simulink model "seguimiento_lmi"  (R2021a)
settings: Solver=VariableStepAuto  StartTime=0.0  StopTime=10.0  RelTol=1e-3
settings Model: Creator=jmata  LastModifiedBy=jmata

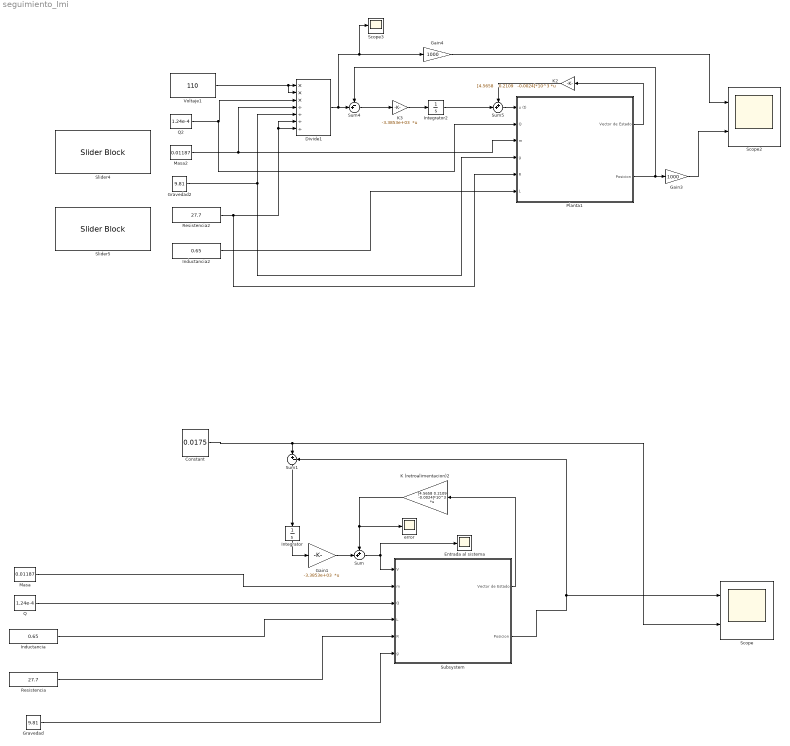
== system seguimiento_lmi ==
  Constant : Constant  Value=0.0175
  Divide1 : Product  Inputs=***////
  Entrada al sistema : Scope
  Gain1 : Gain  Gain=-3.3853e+03  Multiplication=Matrix(K*u)
  Gain3 : Gain  Gain=1000
  Gain4 : Gain  Gain=1000
  Gravedad : Constant  Value=9.81
  Gravedad2 : Constant  Value=9.81
  Inductancia : Constant  Value=0.65  VectorParams1D=off
  Inductancia2 : Constant  Value=0.65
  Integrator : Integrator
  Integrator2 : Integrator
  K (retroalimentacion)2 : Gain  Gain="[4.5658    0.2109   -0.0024]*10^3"  Multiplication=Matrix(K*u)
  K2 : Gain  Gain="[4.5658    0.2109   -0.0024]*10^3"  Multiplication=Matrix(K*u)
  K3 : Gain  Gain=-3.3853e+03  Multiplication=Matrix(K*u)
  Masa : Constant  Value=0.01187
  Masa2 : Constant  Value=0.01187
  Planta1 : Subsystem
  Q : Constant  Value=1.24e-4
  Q2 : Constant  Value=1.24e-4
  Resistencia : Constant  Value=27.7
  Resistencia2 : Constant  Value=27.7
  Scope : Scope  NumInputPorts=2
  Scope2 : Scope  NumInputPorts=2
  Scope3 : Scope
  Slider4 : SliderBlock  ScaleMin=25  ScaleMax=30
  Slider5 : SliderBlock  ScaleMin=0.585  ScaleMax=0.715
  Subsystem : Subsystem
  Sum : Sum  Inputs=++|
  Sum1 : Sum  Inputs=|+-
  Sum4 : Sum  Inputs=-+|
  Sum5 : Sum  Inputs=++|
  Voltaje1 : Constant  Value=110
  error : Scope
  wires:
  Constant/1 -> Scope/2, Sum1/1
  Gravedad/1 -> Subsystem/6(g)
  Masa/1 -> Subsystem/2(m)
  Inductancia/1 -> Subsystem/4(L)
  Sum1/1 -> Integrator/1
  Gain1/1 -> Sum/2
  Integrator/1 -> Gain1/1
  Resistencia/1 -> Subsystem/5(R)
  Subsystem/2(Posicion) -> Sum1/2, Scope/1
  Sum/1 -> Subsystem/1(V), Entrada al sistema/1
  Q/1 -> Subsystem/3(Q)
  Subsystem/1(Vector de Estado) -> K (retroalimentacion)2/1
  K (retroalimentacion)2/1 -> Sum/1, error/1
  Gain4/1 -> Scope2/1
  Divide1/1 -> Sum4/2, Scope3/1, Gain4/1
  Q2/1 -> Planta1/2(Q), Divide1/3
  Gravedad2/1 -> Divide1/5, Planta1/4(g)
  Gain3/1 -> Scope2/2
  Voltaje1/1 -> Divide1/2, Divide1/1
  Sum5/1 -> Planta1/1(u (t))
  Planta1/2(Posicion) -> Gain3/1, Sum4/1
  Masa2/1 -> Planta1/3(m), Divide1/4
  Planta1/1(Vector de Estado) -> K2/1
  Sum4/1 -> K3/1
  K2/1 -> Sum5/1
  K3/1 -> Integrator2/1
  Resistencia2/1 -> Divide1/7, Divide1/6, Planta1/5(R)
  Integrator2/1 -> Sum5/2
  Inductancia2/1 -> Planta1/6(L)

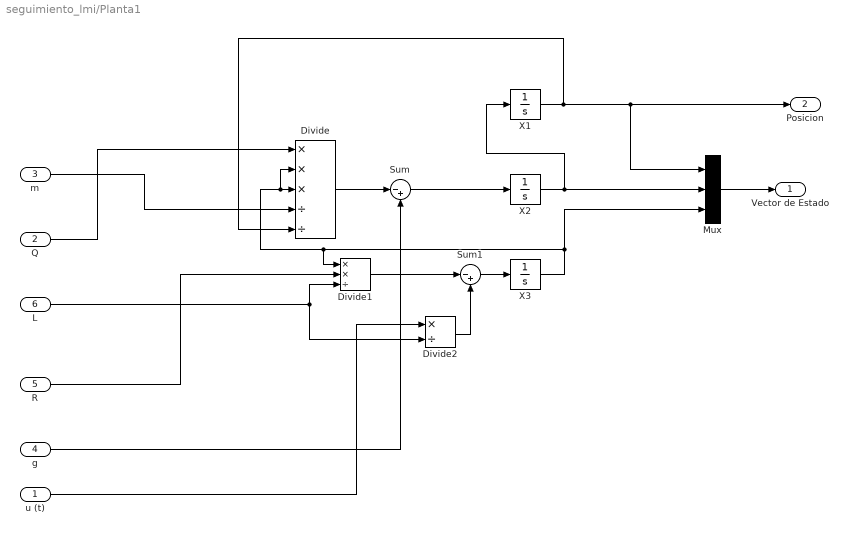
== system seguimiento_lmi/Planta1 ==
  u (t) : Inport
  Q : Inport  Port=2
  m : Inport  Port=3
  g : Inport  Port=4
  R : Inport  Port=5
  L : Inport  Port=6
  Divide : Product  Inputs=***//
  Divide1 : Product  Inputs=**/
  Divide2 : Product  Inputs=*/
  Mux : Mux  Inputs=3
  Sum : Sum  Inputs=|-+
  Sum1 : Sum  Inputs=|-+
  X1 : Integrator  InitialCondition=14.79e-3
  X2 : Integrator
  X3 : Integrator  InitialCondition=110/27.7
  Vector de Estado : Outport
  Posicion : Outport  Port=2
  wires:
  Divide/1 -> Sum/1
  Sum/1 -> X2/1
  L/1 -> Divide2/2, Divide1/3
  Sum1/1 -> X3/1
  X3/1 -> Mux/3, Divide1/1, Divide/2, Divide/3
  Divide2/1 -> Sum1/2
  X1/1 -> Posicion/1, Mux/1, Divide/5
  X2/1 -> Mux/2, X1/1
  g/1 -> Sum/2
  Divide1/1 -> Sum1/1
  m/1 -> Divide/4
  Q/1 -> Divide/1
  Mux/1 -> Vector de Estado/1
  R/1 -> Divide1/2
  u (t)/1 -> Divide2/1

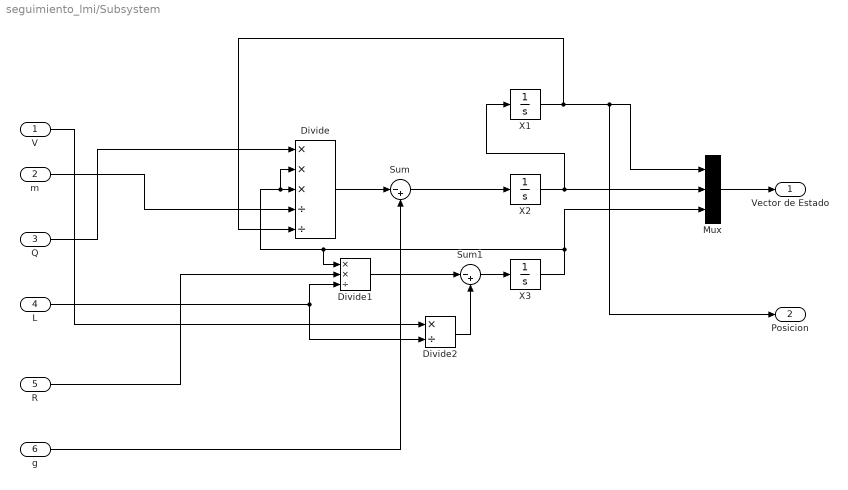
== system seguimiento_lmi/Subsystem ==
  V : Inport
  m : Inport  Port=2
  Q : Inport  Port=3
  L : Inport  Port=4
  R : Inport  Port=5
  g : Inport  Port=6
  Divide : Product  Inputs=***//
  Divide1 : Product  Inputs=**/
  Divide2 : Product  Inputs=*/
  Mux : Mux  Inputs=3
  Sum : Sum  Inputs=|-+
  Sum1 : Sum  Inputs=|-+
  X1 : Integrator  InitialCondition=0.0110
  X2 : Integrator
  X3 : Integrator  InitialCondition=3.82
  Vector de Estado : Outport
  Posicion : Outport  Port=2
  wires:
  Divide/1 -> Sum/1
  Sum/1 -> X2/1
  L/1 -> Divide2/2, Divide1/3
  Sum1/1 -> X3/1
  X3/1 -> Mux/3, Divide1/1, Divide/2, Divide/3
  Divide2/1 -> Sum1/2
  X1/1 -> Posicion/1, Mux/1, Divide/5
  X2/1 -> Mux/2, X1/1
  g/1 -> Sum/2
  Divide1/1 -> Sum1/1
  m/1 -> Divide/4
  Q/1 -> Divide/1
  Mux/1 -> Vector de Estado/1
  R/1 -> Divide1/2
  V/1 -> Divide2/1
